simulink model "model"  (Simulink 10.3)
settings: Solver=VariableStepAuto  StartTime=0.0  StopTime=Tf  FixedStep=0.01  RelTol=1e-3  EnableMultiTasking=on
model workspace (MAT data in the model file):
  Kd = 10
  Ki = 1
  Kp : num (value not decoded)
values from neighbouring files (symbols this model uses):
  g = 9.8    [init_cc.m]
  m = 1000    [init_cc.m]
undefined symbols (not defined in the file or in its folder): a1, a2, a3, a4, a5, b1, b2, b3, Kf, Km
undefined symbols (not defined in the file): max_rob, phi_qsiso
libraries: simulink x2, rllib x1
settings Model: Creator=Felipe Vargas  LastModifiedBy=nikhil  MultithreadedSim=on
settings SolverCC: AutoInsertRateTranBlk=on
settings DataIOCC: LimitDataPoints=on  SignalLoggingSaveFormat=Dataset  ReturnWorkspaceOutputs=on
settings OptimizationCC: ExpressionDepthLimit=128
settings DebuggingCC: UnderspecifiedInitializationDetection=Simplified  MergeDetectMultiDrivingBlocksExec=error  FcnCallInpInsideContextMsg=error  StateNameClashWarn=none
settings GRTTargetCC: CombineOutputUpdateFcns=on  GRTInterface=off

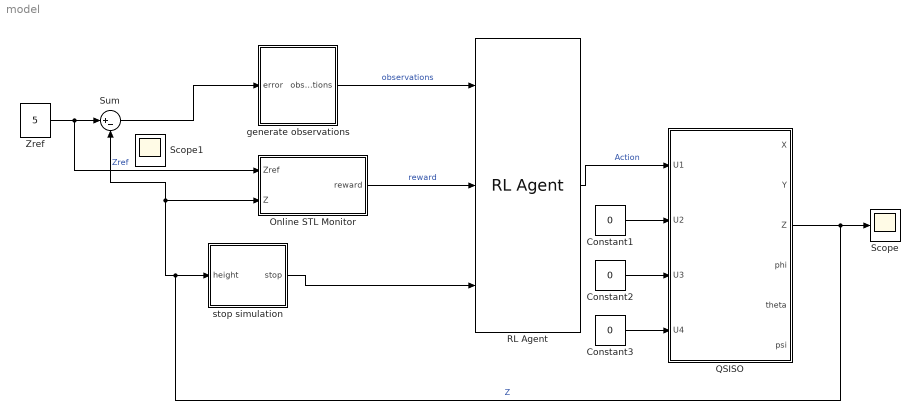
== system model ==
  Constant1 : Constant  Value=0
  Constant2 : Constant  Value=0
  Constant3 : Constant  Value=0
  Online STL Monitor : Subsystem
  QSISO : Subsystem
  RL Agent : rllib/RL Agent  Agent=agent  ExternalActionAsInput=off  ProvideCumRwd=off  TreatAsDirectFeedthrough=on
  Scope : Scope
  Sum : Sum  Inputs=|+-
  Zref : Constant  Value=5
  generate observations : Subsystem
  stop simulation : Subsystem
  Scope1 : Scope
  wires:
  Zref/1 -> Online STL Monitor/1(Zref), Sum/1  "Zref"
  Constant1/1 -> QSISO/2(U2)
  Constant2/1 -> QSISO/3(U3)
  Constant3/1 -> QSISO/4(U4)
  RL Agent/1 -> QSISO/1(U1)  "Action"
  stop simulation/1(stop) -> RL Agent/3
  QSISO/3(Z) -> Scope/1, stop simulation/1(height), Online STL Monitor/2(Z), Sum/2  "Z"
  Online STL Monitor/1(reward) -> RL Agent/2  "reward"
  generate observations/1(observations) -> RL Agent/1  "observations"
  Sum/1 -> generate observations/1(error)

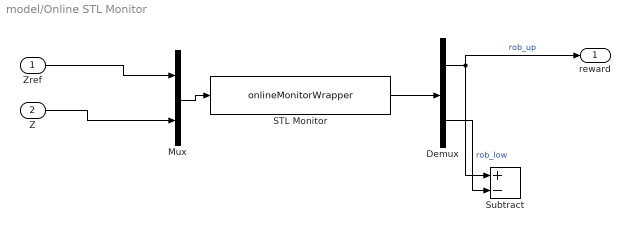
== system model/Online STL Monitor ==
  Zref : Inport
  Z : Inport  Port=2
  Demux : Demux  Outputs=2
  Mux : Mux  Inputs=2
  STL Monitor : S-Function  FunctionName=onlineMonitorWrapper  Parameters=SignalNames, STLString, MaxRob,RefreshRate  SFunctionDeploymentMode=off  EnableBusSupport=off  mask(STL Monitor){SignalNames='Zref,Z', STLString=phi_qsiso, MaxRob=max_rob, RefreshRate=0.1}
      mask prompts: SignalNames "Signal names"; STLString "String For STL formula"; MaxRob "Maximum robustness"; RefreshRate "Refresh Rate"
      mask help:
      | Monitor an STL Formula on input signal. Takes two parameters: a string with
      | comma separated identifiers for the input signals, (ex: 'x1,x2,y'), and a
      | string for the formula (ex: 'alw_[0, 50] (x1[t]>0 => y[t] >0)'). Outputs a
      | two dimensional signal bounding the satisfaction of the formula.
      mask Display: fprintf('%s', STLString)
  Subtract : Sum  Inputs=+-
  reward : Outport
  wires:
  Mux/1 -> STL Monitor/1
  STL Monitor/1 -> Demux/1
  Demux/2 -> Subtract/2  "rob_low"
  Demux/1 -> reward/1, Subtract/1  "rob_up"
  Zref/1 -> Mux/1
  Z/1 -> Mux/2

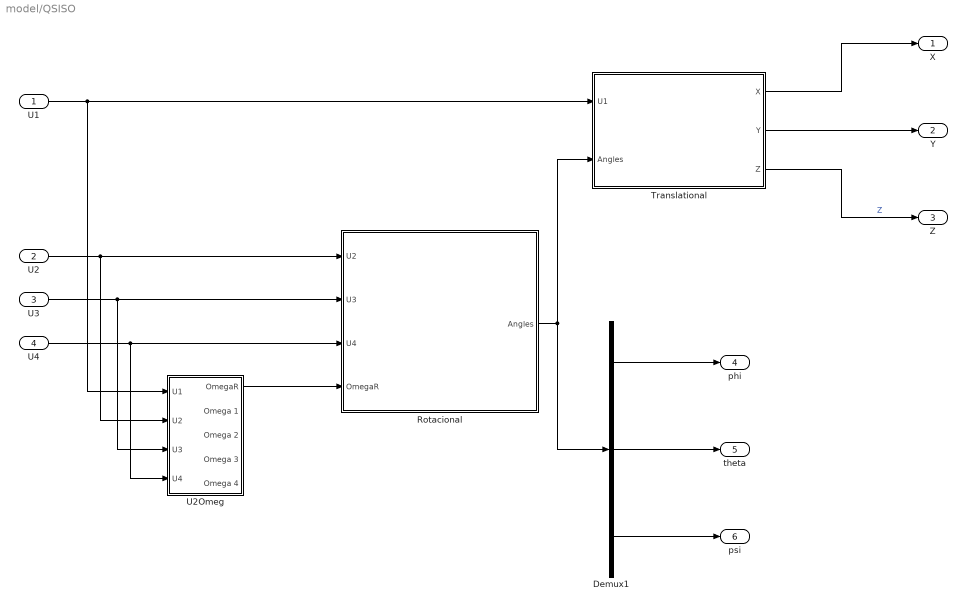
== system model/QSISO ==
  U1 : Inport
  U2 : Inport  Port=2
  U3 : Inport  Port=3
  U4 : Inport  Port=4
  Demux1 : Demux  Outputs=3
  Rotacional : Subsystem
  Translational : Subsystem
  U2Omeg : Subsystem
  X : Outport
  Y : Outport  Port=2
  Z : Outport  Port=3
  phi : Outport  Port=4
  theta : Outport  Port=5
  "psi " : Outport  Port=6
  wires:
  Rotacional/1(Angles) -> Translational/2(Angles), Demux1/1
  Demux1/1 -> phi/1
  Demux1/2 -> theta/1
  Demux1/3 -> "psi "/1
  Translational/1(X) -> X/1
  Translational/3(Z) -> Z/1  "Z"
  Translational/2(Y) -> Y/1
  U2/1 -> U2Omeg/2("U2 "), Rotacional/1(U2)
  U1/1 -> Translational/1(U1), U2Omeg/1("U1 ")
  U4/1 -> U2Omeg/4("U4 "), Rotacional/3(U4)
  U3/1 -> U2Omeg/3("U3 "), Rotacional/2(U3)
  U2Omeg/1(OmegaR) -> Rotacional/4(OmegaR)

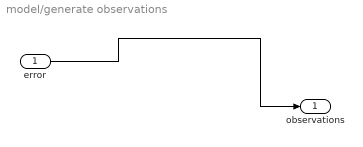
== system model/generate observations ==
  error : Inport
  observations : Outport  VectorParamsAs1DForOutWhenUnconnected=off
  wires:
  error/1 -> observations/1

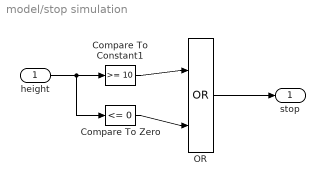
== system model/stop simulation ==
  height : Inport
  Compare To Constant1 : simulink/Logic and Bit Operations/Compare To Constant  relop=>=  const=10  OutDataTypeStr=boolean
  Compare To Zero : simulink/Logic and Bit Operations/Compare To Zero  relop=<=  OutDataTypeStr=boolean
  OR : Logic  Operator=OR  IconShape=distinctive  AllPortsSameDT=off  OutDataTypeStr=boolean
  stop : Outport  VectorParamsAs1DForOutWhenUnconnected=off
  wires:
  Compare To Zero/1 -> OR/2
  OR/1 -> stop/1
  height/1 -> Compare To Zero/1, Compare To Constant1/1
  Compare To Constant1/1 -> OR/1

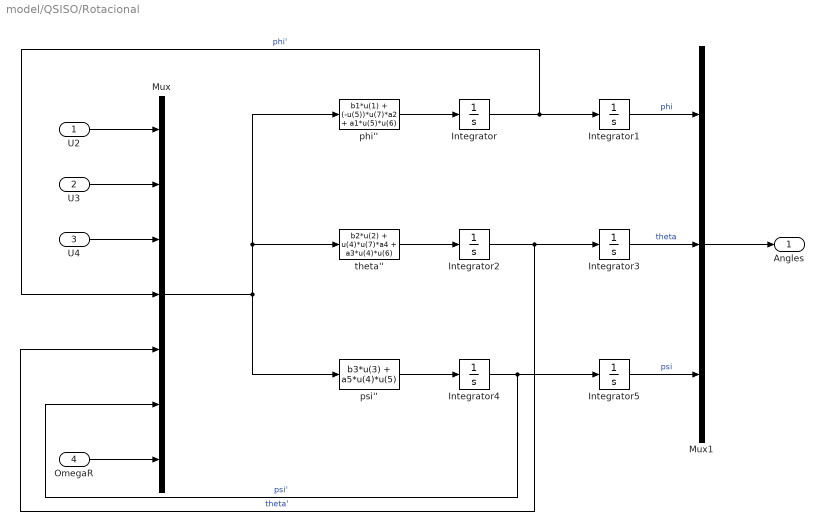
== system model/QSISO/Rotacional ==
  U2 : Inport
  U3 : Inport  Port=2
  U4 : Inport  Port=3
  OmegaR : Inport  Port=4
  Integrator{,1..5} (6 alike) : Integrator
  Mux : Mux  Inputs=7
  Mux1 : Mux  Inputs=3
  phi'' : Fcn  Expr=b1*u(1) + (-u(5))*u(7)*a2 + a1*u(5)*u(6)
  psi'' : Fcn  Expr=b3*u(3) + a5*u(4)*u(5)
  theta'' : Fcn  Expr=b2*u(2) + u(4)*u(7)*a4 + a3*u(4)*u(6)
  Angles : Outport
  wires:
  U2/1 -> Mux/1
  U3/1 -> Mux/2
  U4/1 -> Mux/3
  phi''/1 -> Integrator/1
  Integrator/1 -> Mux/4, Integrator1/1  "phi'"
  Mux/1 -> psi''/1, theta''/1, phi''/1
  theta''/1 -> Integrator2/1
  Integrator2/1 -> Mux/5, Integrator3/1  "theta'"
  psi''/1 -> Integrator4/1
  Integrator4/1 -> Mux/6, Integrator5/1  "psi'"
  Integrator1/1 -> Mux1/1  "phi"
  Integrator3/1 -> Mux1/2  "theta"
  Mux1/1 -> Angles/1
  Integrator5/1 -> Mux1/3  "psi"
  OmegaR/1 -> Mux/7

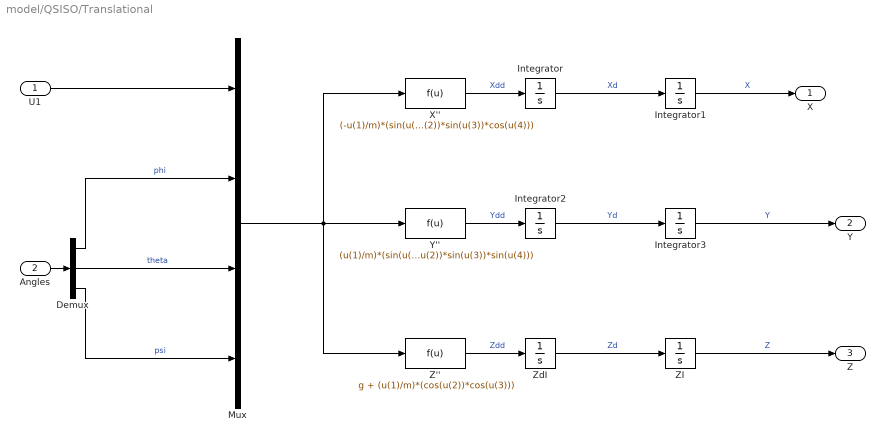
== system model/QSISO/Translational ==
  U1 : Inport
  Angles : Inport  Port=2
  Demux : Demux  Outputs=3
  Integrator{,1..3} (4 alike) : Integrator
  Mux : Mux
  X'' : Fcn  Expr=(-u(1)/m)*(sin(u(2))*sin(u(4)) + cos(u(2))*sin(u(3))*cos(u(4)))
  Y'' : Fcn  Expr=(u(1)/m)*(sin(u(2))*cos(u(4)) - cos(u(2))*sin(u(3))*sin(u(4)))
  Z'' : Fcn  Expr=g + (u(1)/m)*(cos(u(2))*cos(u(3)))
  ZI : Integrator  InitialCondition=4.2218  LowerSaturationLimit=0
  ZdI : Integrator  LowerSaturationLimit=0
  X : Outport
  Y : Outport  Port=2
  Z : Outport  Port=3
  wires:
  X''/1 -> Integrator/1  "Xdd"
  Integrator/1 -> Integrator1/1  "Xd"
  Angles/1 -> Demux/1
  Mux/1 -> Z''/1, Y''/1, X''/1
  U1/1 -> Mux/1
  Demux/1 -> Mux/2  "phi"
  Demux/2 -> Mux/3  "theta"
  Demux/3 -> Mux/4  "psi"
  Y''/1 -> Integrator2/1  "Ydd"
  Integrator2/1 -> Integrator3/1  "Yd"
  Integrator3/1 -> Y/1  "Y"
  Z''/1 -> ZdI/1  "Zdd"
  ZdI/1 -> ZI/1  "Zd"
  ZI/1 -> Z/1  "Z"
  Integrator1/1 -> X/1  "X"

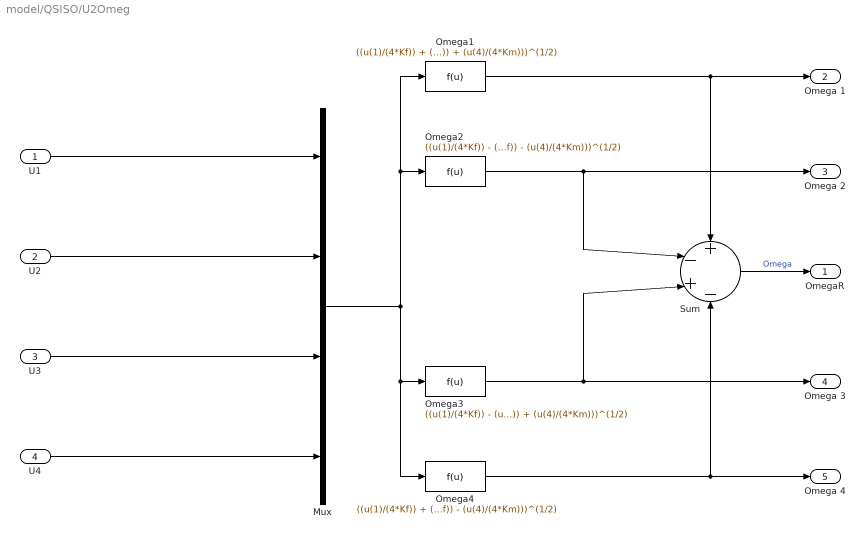
== system model/QSISO/U2Omeg ==
  "U1 " : Inport
  "U2 " : Inport  Port=2
  "U3 " : Inport  Port=3
  "U4 " : Inport  Port=4
  Mux : Mux
  Omega1 : Fcn  Expr=((u(1)/(4*Kf)) + (u(3)/(2*Kf)) + (u(4)/(4*Km)))^(1/2)
  Omega2 : Fcn  Expr=((u(1)/(4*Kf)) - (u(2)/(2*Kf)) - (u(4)/(4*Km)))^(1/2)
  Omega3 : Fcn  Expr=((u(1)/(4*Kf)) - (u(3)/(2*Kf)) + (u(4)/(4*Km)))^(1/2)
  Omega4 : Fcn  Expr=((u(1)/(4*Kf)) + (u(2)/(2*Kf)) - (u(4)/(4*Km)))^(1/2)
  Sum : Sum  Inputs=+-+-
  OmegaR : Outport
  Omega 1 : Outport  Port=2
  Omega 2 : Outport  Port=3
  Omega 3 : Outport  Port=4
  Omega 4 : Outport  Port=5
  wires:
  Omega2/1 -> Sum/2, Omega 2/1
  Omega1/1 -> Sum/1, Omega 1/1
  Omega3/1 -> Sum/3, Omega 3/1
  Mux/1 -> Omega2/1, Omega1/1, Omega4/1, Omega3/1
  Omega4/1 -> Omega 4/1, Sum/4
  "U4 "/1 -> Mux/4
  "U3 "/1 -> Mux/3
  "U2 "/1 -> Mux/2
  "U1 "/1 -> Mux/1
  Sum/1 -> OmegaR/1  "Omega"
